simulink model "D53_LKA_Software"  (R2018b)
settings: Solver=ode3  StartTime=0.0  StopTime=10.0  FixedStep=0.01  RelTol=1e-3  EnableMultiTasking=on
model workspace (MAT data in the model file):
  MCOS : class17 (value not decoded)
  MCOS : class17 (value not decoded)
  MCOS : class17 (value not decoded)
  MCOS : class17 (value not decoded)
  MCOS : class17 (value not decoded)
  MCOS : class17 (value not decoded)
  MCOS : class17 (value not decoded)
  MCOS : class17 (value not decoded)
  MCOS : class17 (value not decoded)
  MCOS : class17 (value not decoded)
  MCOS : class17 (value not decoded)
  MCOS : class17 (value not decoded)
  MCOS : class17 (value not decoded)
  MCOS : class17 (value not decoded)
  MCOS : class17 (value not decoded)
  MCOS : class17 (value not decoded)
  MCOS : class17 (value not decoded)
  MCOS : class17 (value not decoded)
  MCOS : class17 (value not decoded)
  MCOS : class17 (value not decoded)
  MCOS : class17 (value not decoded)
  MCOS : class17 (value not decoded)
  MCOS : class17 (value not decoded)
  MCOS : class17 (value not decoded)
  MCOS : class17 (value not decoded)
  MCOS : class17 (value not decoded)
  MCOS : class17 (value not decoded)
  MCOS : class17 (value not decoded)
  MCOS : class17 (value not decoded)
  MCOS : class17 (value not decoded)
  MCOS : class17 (value not decoded)
  MCOS : class17 (value not decoded)
  MCOS : class17 (value not decoded)
  MCOS : class17 (value not decoded)
  MCOS : class17 (value not decoded)
  MCOS : class17 (value not decoded)
  MCOS : class17 (value not decoded)
  MCOS : class17 (value not decoded)
  MCOS : class17 (value not decoded)
  MCOS : class17 (value not decoded)
  MCOS : class17 (value not decoded)
  MCOS : class17 (value not decoded)
  MCOS : class17 (value not decoded)
  MCOS : class17 (value not decoded)
  MCOS : class17 (value not decoded)
  MCOS : class17 (value not decoded)
  MCOS : class17 (value not decoded)
  MCOS : class17 (value not decoded)
  MCOS : class17 (value not decoded)
  MCOS : class17 (value not decoded)
  MCOS : class17 (value not decoded)
  MCOS : class17 (value not decoded)
  MCOS : class17 (value not decoded)
  MCOS : class17 (value not decoded)
  MCOS : class17 (value not decoded)
  MCOS : class17 (value not decoded)
  MCOS : class17 (value not decoded)
  MCOS : class17 (value not decoded)
  MCOS : class17 (value not decoded)
  MCOS : class17 (value not decoded)
  MCOS : class17 (value not decoded)
  MCOS : class17 (value not decoded)
  MCOS : class17 (value not decoded)
  MCOS : class17 (value not decoded)
  MCOS : class17 (value not decoded)
  MCOS : class17 (value not decoded)
  MCOS : class17 (value not decoded)
  MCOS : class17 (value not decoded)
  MCOS : class17 (value not decoded)
  MCOS : class17 (value not decoded)
  MCOS : class17 (value not decoded)
  MCOS : class17 (value not decoded)
  MCOS : class17 (value not decoded)
  MCOS : class17 (value not decoded)
  MCOS : class17 (value not decoded)
  MCOS : class17 (value not decoded)
  MCOS : class17 (value not decoded)
  MCOS : class17 (value not decoded)
  MCOS : class17 (value not decoded)
  MCOS : class17 (value not decoded)
  MCOS : class17 (value not decoded)
  MCOS : class17 (value not decoded)
  MCOS : class17 (value not decoded)
  MCOS : class17 (value not decoded)
  MCOS : class17 (value not decoded)
  MCOS : class17 (value not decoded)
  MCOS : class17 (value not decoded)
  MCOS : class17 (value not decoded)
  MCOS : class17 (value not decoded)
undefined symbols (not defined in the file or in its folder): LKA_CarWidth, LKA_SampleTime, LKA_StrRatio_C, LKA_Veh2CamL_C, LKA_Veh2CamW_C, LKA_WhlBaseL_C, LL_CompSWA_C, LL_CrvtPrvwT_C, LL_DesDvt_C, LL_DvtComp_C, LL_DvtPrvwT_C, LL_DvtSpdDet_vDvtSpdMin_C, LL_HdAgExT_C, LL_HdAgPrvwT_C, LL_LAccMax_C, LL_LAccRMax_C, LL_LDW_EarliestWarnLine_C, LL_LDW_LatestWarnLine_C, LL_LDWS_SUPPRESS_HEADING, LL_LFClb_TFC_DiffCtlBalance, LL_LFClb_TFC_DiffCtrlMaxSWA, LL_LFClb_TFC_DiffCtrlRatio, LL_LFClb_TFC_facmGainLutGain1_C, LL_LFClb_TFC_facmGainLutGain2_C, LL_LFClb_TFC_facmIntegRatio, LL_LFClb_TFC_facmKlat_C, LL_LFClb_TFC_FfCtlRatio_C, LL_LFClb_TFC_phiIntegCtlMaxSWA_C, LL_LFClb_TFC_tiKlatPrvwT_C, LL_LFClb_TFC_vGainLutVehSpdLwr_C, LL_LFClb_TFC_vGainLutVehSpdUpr_C, LL_LKA_EarliestWarnLine_C, LL_LKA_LatestWarnLine_C, LL_LKAExPrcs_ExitC0Dvt, LL_LKAExPrcs_ExitC0Swt, LL_LKAExPrcs_tiExitTime1, LL_LKAExPrcs_tiExitTime2, LL_LKAExPrcs_tiExitTime3, LL_LKAS_OUT_OF_CONTROL_LAT_VEL, LL_LKAS_OUT_OF_CONTROL_TTLC, LL_LKASWASyn_M0, LL_LKASWASyn_M1, LL_LKASWASyn_M2, LL_LKASWASyn_M3K, LL_LKASWASyn_SWAaddMax, LL_LKASWASyn_T2, LL_LKASWASyn_tiTrqSwaRtTime, LL_LKASWASyn_tiTrqSwaTime, LL_LKASWASyn_TrqMax, LL_LKASWASyn_TrqSwaAddSwt, LL_LKASWASyn_TrqSwaRateDiff, LL_LSpdCompT_C, LL_lStpLngth_C, LL_MAX_DELAY_EPSSTAR_TIME, LL_MAX_DRIVER_TORQUE_DISABLE, LL_MAX_DRIVER_TORQUE_ENABLE, LL_MAX_LANE_WIDTH_DISABLE, LL_MAX_LANE_WIDTH_ENABLE, LL_MAX_LAT_ACC_DISABLE, LL_MAX_LAT_ACC_ENABLE ... (+30)
libraries: simulink x167, canmsglib x52, dspstat3 x3, simulink_extras x1
(part 4 of 21)

== system D53_LKA_Software/CAN Monitor (CANMon)/Subsystem1 ==
  In1 : Inport
  In2 : Inport  Port=2
  Abs : Abs
  Add : Sum  OutDataTypeStr=single
  Compare To Zero : simulink/Logic and Bit Operations/Compare To Zero  relop===  OutDataTypeStr=boolean
  Constant : Constant  OutDataTypeStr=single  SampleTime=-1
  Constant1 : Constant  Value=0.000000001  OutDataTypeStr=single  SampleTime=-1
  Divide : Product  Inputs=*/  OutDataTypeStr=single
  Switch : Switch  Criteria=u2 ~= 0
  Out1 : Outport
  wires:
  Add/1 -> Abs/1
  In1/1 -> Add/1
  Compare To Zero/1 -> Switch/2
  In2/1 -> Add/2
  Constant/1 -> Divide/1
  Switch/1 -> Divide/2
  Constant1/1 -> Switch/1
  Divide/1 -> Out1/1
  Abs/1 -> Switch/3, Compare To Zero/1

== system D53_LKA_Software/LL/Fault_Diagnostic ==
  bsInInfo : Inport
  Bus Creator : BusCreator  Inputs=2
  Bus Creator1 : BusCreator  Inputs=12
  Bus Selector3 : BusSelector  OutputSignals=DTC_Indicator.LKAS_BSWDTC_Status
  Bus Selector4 : BusSelector  OutputSignals=bsVehMovInfo.ESC_VehSpd_Valid,bsEPSInfo.EPS_LKA_State,bsEPSInfo.EPS_Error_State,bsEPSInfo.SAS_Clb_State,bsEPSInfo.SAS_Trim_State,bsSWAInfo.SWS_Fault_Code,bsSWAInfo.SAS_In_Status,bsPTState.TCU_ActualGear,bsEPSInfo.EPS_TrqLim_State,bsEPSInfo.EPS_Trq_State,bsVehMovInfo.ESC_LatAcc_Valid,bsVehMovInfo.ESC_YawRate_Valid,bsVehMovInfo.ESC_LonAcc_Valid
  Compare To Constant26 : simulink/Logic and Bit Operations/Compare To Constant  relop=~=  const=1  OutDataTypeStr=boolean
  Compare To Constant27 : simulink/Logic and Bit Operations/Compare To Constant  relop===  const=4  OutDataTypeStr=boolean
  Compare To Constant{28,30,36..39} (6 alike) : simulink/Logic and Bit Operations/Compare To Constant  relop===  const=1  OutDataTypeStr=boolean
  Compare To Constant29 : simulink/Logic and Bit Operations/Compare To Constant  relop===  const=0  OutDataTypeStr=boolean
  Compare To Constant31 : simulink/Logic and Bit Operations/Compare To Constant  relop===  const=2  OutDataTypeStr=boolean
  Compare To Constant32 : simulink/Logic and Bit Operations/Compare To Constant  relop=~=  const=0  OutDataTypeStr=boolean
  Compare To Constant33 : simulink/Logic and Bit Operations/Compare To Constant  relop=~=  const=1  OutDataTypeStr=boolean
  Compare To Constant34 : simulink/Logic and Bit Operations/Compare To Constant  relop=>  const=3  OutDataTypeStr=boolean
  Compare To Constant35 : simulink/Logic and Bit Operations/Compare To Constant  relop===  const=0  OutDataTypeStr=boolean
  Logical Operator5 : Logic  Operator=OR  AllPortsSameDT=off  OutDataTypeStr=boolean
  Logical Operator6 : Logic  Operator=OR  AllPortsSameDT=off  OutDataTypeStr=boolean
  bsSignalFault : Outport
  wires:
  Bus Creator/1 -> bsSignalFault/1
  Bus Selector3/1 -> Bus Creator/1  "<LKAS_BSWDTC_Status>"
  bsInInfo/1 -> Bus Selector4/1, Bus Selector3/1
  Bus Selector4/1 -> Compare To Constant26/1  "<ESC_VehSpd_Valid>"
  Compare To Constant26/1 -> Bus Creator1/1  "Event_FaulVehSpeed"
  Bus Selector4/2 -> Compare To Constant27/1  "<EPS_LKA_State>"
  Bus Selector4/4 -> Compare To Constant29/1  "<SAS_Clb_State>"
  Compare To Constant29/1 -> Bus Creator1/4  "Event_FaulSASClb"
  Bus Selector4/5 -> Compare To Constant30/1  "<SAS_Trim_State>"
  Bus Selector4/6 -> Compare To Constant32/1  "<SWS_Fault_Code>"
  Bus Selector4/7 -> Compare To Constant33/1  "<SAS_In_Status>"
  Bus Selector4/8 -> Compare To Constant34/1  "<TCU_ActualGear>"
  Bus Selector4/9 -> Compare To Constant35/1  "<EPS_TrqLim_State>"
  Bus Selector4/10 -> Compare To Constant36/1  "<EPS_Trq_State>"
  Bus Selector4/11 -> Compare To Constant37/1  "<ESC_LatAcc_Valid>"
  Bus Selector4/12 -> Compare To Constant38/1  "<ESC_YawRate_Valid>"
  Bus Selector4/13 -> Compare To Constant39/1  "<ESC_LonAcc_Valid>"
  Compare To Constant30/1 -> Bus Creator1/5  "Event_FaulSASTrim"
  Compare To Constant31/1 -> Logical Operator5/2
  Compare To Constant28/1 -> Logical Operator5/1
  Bus Selector4/3 -> Compare To Constant31/1, Compare To Constant28/1  "<EPS_Error_State>"
  Compare To Constant32/1 -> Logical Operator6/1
  Compare To Constant33/1 -> Logical Operator6/2
  Compare To Constant35/1 -> Bus Creator1/8  "Event_FaulTrqLim"
  Compare To Constant34/1 -> Bus Creator1/7  "Event_FaulTCUGear"
  Compare To Constant36/1 -> Bus Creator1/9  "Event_FaulEPSTrqSt"
  Compare To Constant37/1 -> Bus Creator1/10  "Event_FaulLatAcc"
  Compare To Constant38/1 -> Bus Creator1/11  "Event_FaulYawRate"
  Compare To Constant39/1 -> Bus Creator1/12  "Event_FaulLonAcc"
  Bus Creator1/1 -> Bus Creator/2  "LKAS_ASWDTC_Status"
  Compare To Constant27/1 -> Bus Creator1/2  "Event_FaulEPSLKASt"
  Logical Operator5/1 -> Bus Creator1/3  "Event_FaulETATDA"
  Logical Operator6/1 -> Bus Creator1/6  "Event_FaulSWS"

== system D53_LKA_Software/LL/Human Machine Interface (HMI) ==
  HMI_stDACmode : Inport
  HMI_LDWWarn : Inport  Port=2
  HMI_LKA_STATE : Inport  Port=3
  HMI_LDW_STATE : Inport  Port=4
  HMI_R0_Quality : Inport  Port=5
  HMI_L0_Quality : Inport  Port=6
  HMI_EPSInfo : Inport  Port=7
  HMI_camera_common_fault : Inport  Port=8
  HMI_Front_Camera_Blocked : Inport  Port=9
  HMI_stFaultCSyn : Inport  Port=10
  Bus Creator2 : BusCreator  Inputs=7
  Cast To Single{,1..6} (7 alike) : DataTypeConversion  OutDataTypeStr=uint8
  HMI_Popup_Status : MATLAB Function  TreatAsAtomicUnit=on
  Hands_off_warning : MATLAB Function  TreatAsAtomicUnit=on
  LDW_Flag : MATLAB Function  TreatAsAtomicUnit=on
  LDW_Status_Display : MATLAB Function  TreatAsAtomicUnit=on
  LKA_Status_Display : MATLAB Function  TreatAsAtomicUnit=on
  LKA_action_indication : MATLAB Function  TreatAsAtomicUnit=on
  Subsystem : Subsystem
  Vehicle_Lane_Display : MATLAB Function  TreatAsAtomicUnit=on
  HMI_LDWLKA : Outport
  wires:
  HMI_LKA_STATE/1 -> Vehicle_Lane_Display/2(LKA_STATE), LKA_Status_Display/2(LKA_STATE), LDW_Flag/2(HMI_LKA_STATE), HMI_Popup_Status/2(LKA_STATE), LKA_action_indication/2(LKA_STATE)  "HMI_LKA_STATE"
  HMI_LDW_STATE/1 -> Subsystem/1(LDW_STATE), Vehicle_Lane_Display/3(LDW_STATE), LDW_Status_Display/2(LDW_STATE)  "HMI_LDW_STATE"
  Hands_off_warning/1(Hands_off_warning) -> Cast To Single4/1  "Hands_off_warning"
  LDW_Status_Display/1(LDW_Status_Display) -> Cast To Single1/1  "LDW_Status_Display"
  HMI_stFaultCSyn/1 -> HMI_Popup_Status/6(stFaultCSyn)  "HMI_stFaultCSyn"
  Bus Creator2/1 -> HMI_LDWLKA/1
  HMI_L0_Quality/1 -> Vehicle_Lane_Display/5(L0_Quality)  "HMI_L0_Quality"
  HMI_Popup_Status/1(HMI_Popup_Status) -> Cast To Single6/1  "HMI_Popup_Status"
  LKA_Status_Display/1(LKA_Status_Display) -> Cast To Single2/1  "LKA_Status_Display"
  HMI_stDACmode/1 -> Vehicle_Lane_Display/1(stDACmode), LDW_Status_Display/1(stDACmode), HMI_Popup_Status/1(stDACmode), LKA_action_indication/1(stDACmode), LDW_Flag/1(HMI_stDACmode), LKA_Status_Display/1(stDACmode)  "HMI_stDACmode"
  LDW_Flag/1(LDW_Flag) -> Cast To Single3/1  "LDW_Flag"
  HMI_Front_Camera_Blocked/1 -> HMI_Popup_Status/5(Front_Camera_Blocked)  "HMI_Front_Camera_Blocked"
  HMI_R0_Quality/1 -> Vehicle_Lane_Display/4(R0_Quality)  "HMI_R0_Quality"
  HMI_camera_common_fault/1 -> HMI_Popup_Status/4(camera_common_fault)  "HMI_camera_common_fault"
  LKA_action_indication/1(LKA_action_indication) -> Cast To Single5/1  "LKA_action_indication"
  Vehicle_Lane_Display/1(Vehicle_Lane_Display) -> Cast To Single/1  "Vehicle_Lane_Display"
  Cast To Single/1 -> Bus Creator2/1  "Vehicle_Lane_Display"
  Cast To Single1/1 -> Bus Creator2/2  "LDW_Status_Display"
  Cast To Single2/1 -> Bus Creator2/3  "LKA_Status_Display"
  Cast To Single3/1 -> Bus Creator2/4  "LDW_Flag"
  Cast To Single4/1 -> Bus Creator2/5  "Hands_off_warning"
  Cast To Single5/1 -> Bus Creator2/6  "LKA_action_indication"
  Cast To Single6/1 -> Bus Creator2/7  "HMI_Popup_Status"
  HMI_EPSInfo/1 -> Subsystem/2(EPSInfo)  "HMI_EPSInfo"
  Subsystem/1(HandsOff10s) -> HMI_Popup_Status/3(HandsOff)
  Subsystem/2(HandsOff15s) -> Hands_off_warning/1(HandsOff)
  HMI_LDWWarn/1 -> LDW_Flag/3(HMI_LDWWarnInfo)

== system D53_LKA_Software/LL/LL Inputs Mapping ==
  bsInInfo : Inport
  Bus Creator : BusCreator  Inputs=7
  Bus Selector : BusSelector  OutputSignals=bsMP5Info,bsLaneInfo,bsEPSInfo,bsVehMovInfo,bsSWAInfo,bsBCMInfo,bsPTState
  bsBCMInfo : Subsystem
  bsEPSInfo : Subsystem
  bsLaneInfo : Subsystem
  bsMP5Info : Subsystem
  bsPTState : Subsystem
  bsSWAInfo : Subsystem
  bsVehMovInfo : Subsystem
  bsInfo : Outport
  wires:
  bsInInfo/1 -> Bus Selector/1
  Bus Creator/1 -> bsInfo/1
  Bus Selector/2 -> bsLaneInfo/1(bsLaneInfoIn)  "<bsLaneInfo>"
  Bus Selector/3 -> bsEPSInfo/1(bsEPSInfoIn)  "<bsEPSInfo>"
  bsEPSInfo/1(bsEPSInfoOut) -> Bus Creator/3  "bsEPSInfo"
  Bus Selector/4 -> bsVehMovInfo/1(bsVehMovInfoIn)  "<bsVehMovInfo>"
  bsVehMovInfo/1(bsVehMovInfoOut) -> Bus Creator/4  "bsVehMovInfo"
  Bus Selector/5 -> bsSWAInfo/1(bsSWAInfoIn)  "<bsSWAInfo>"
  Bus Selector/6 -> bsBCMInfo/1(bsBCMInfoIn)  "<bsBCMInfo>"
  Bus Selector/1 -> bsMP5Info/1(bsMP5InfoIn)  "<bsMP5Info>"
  bsMP5Info/1(bsMP5InfoOut) -> Bus Creator/1  "bsMP5Info"
  bsBCMInfo/1(bsBCMInfoOut) -> Bus Creator/6  "bsBCMInfo"
  Bus Selector/7 -> bsPTState/1(bsPTStateIn)  "<bsPTState>"
  bsPTState/1(bsPTStateOut) -> Bus Creator/7  "bsPTState"
  bsLaneInfo/1(bsLaneInfoOut) -> Bus Creator/2  "bsLaneInfo"
  bsSWAInfo/1(bsSWAInfoOut) -> Bus Creator/5  "bsSWAInfo"

== system D53_LKA_Software/LL/LL Output (LLOut) ==
  LLOut_bsLLState : Inport
  LLOut_phiSWACmd : Inport  Port=2
  LLOut_bsLLHMI : Inport  Port=3
  LLOut_M : Inport  Port=4
  Bus Creator : BusCreator  Inputs=15
  Bus Selector1 : BusSelector  OutputSignals=LKA_State,DACMode
  Bus Selector2 : BusSelector  OutputSignals=Vehicle_Lane_Display,LDW_Status_Display,LKA_Status_Display,LDW_Flag,Hands_off_warning,LKA_action_indication,HMI_Popup_Status
  Cast To Single : DataTypeConversion  OutDataTypeStr=single
  Cast To Single{2,4..15} (13 alike) : DataTypeConversion  OutDataTypeStr=uint8
  Cast To Single3 : DataTypeConversion  OutDataTypeStr=single
  Compare To Constant : simulink/Logic and Bit Operations/Compare To Constant  relop===  const=4  OutDataTypeStr=boolean
  Compare To Constant1 : simulink/Logic and Bit Operations/Compare To Constant  relop=>  const=0  OutDataTypeStr=boolean
  Constant : Constant  Value=0  OutDataTypeStr=uint8
  Constant1 : Constant  OutDataTypeStr=uint8
  Constant15 : Constant  Value=0  OutDataTypeStr=uint16
  Constant2 : Constant  Value=2  OutDataTypeStr=uint8
  Constant25 : Constant  Value=0  OutDataTypeStr=uint8
  Constant26 : Constant  Value=0  OutDataTypeStr=uint8
  Constant3 : Constant  Value=3  OutDataTypeStr=uint8
  Constant4 : Constant  Value=4  OutDataTypeStr=uint8
  Constant5 : Constant  Value=4  OutDataTypeStr=uint8
  Constant6 : Constant  Value=5  OutDataTypeStr=uint8
  Constant7 : Constant  Value=0  OutDataTypeStr=single
  Multiport Switch : MultiPortSwitch  DataPortOrder=Zero-based contiguous  Inputs=7  zeroidx=on
  Switch : Switch  Criteria=u2 > Threshold
  LL_bsLLOut : Outport
  wires:
  Constant/1 -> Multiport Switch/2
  Constant5/1 -> Multiport Switch/7
  Cast To Single13/1 -> Bus Creator/13  "LKA_Mode_from_Camera"
  Cast To Single11/1 -> Bus Creator/11  "Hands_off_warning"
  Constant25/1 -> Cast To Single14/1  "TJA_HMI_Txt_Disp"
  LLOut_M/1 -> Switch/1
  Bus Selector2/2 -> [LDW_Status_Display]  "<LDW_Status_Display>"
  Cast To Single9/1 -> Bus Creator/9  "HMI_Popup_Status"
  Constant4/1 -> Multiport Switch/6
  Bus Selector2/6 -> [LKA_action_indication]  "<LKA_action_indication>"
  Cast To Single15/1 -> Bus Creator/15  "TJA_status_icon"
  Compare To Constant1/1 -> [LKA_Switch_State]
  LLOut_bsLLState/1 -> Bus Selector1/1
  Constant1/1 -> Multiport Switch/3
  Bus Selector2/1 -> [Vehicle_Lane_Display]  "<Vehicle_Lane_Display>"
  LLOut_bsLLHMI/1 -> Bus Selector2/1
  [EPS_State_Ctl] -> Cast To Single2/1  "EPS_State_Ctl"
  [LKA_Mode_from_Camera] -> Cast To Single13/1  "LKA_Mode_from_Camera"
  Cast To Single12/1 -> Bus Creator/12  "Vehicle_Lane_Display"
  Cast To Single6/1 -> Bus Creator/6  "LDW_Status_Display"
  Constant7/1 -> Switch/3
  Switch/1 -> [Coefficient_toregulate_EPS]  "Coefficient_toregulate_EPS"
  Multiport Switch/1 -> [EPS_State_Ctl], Compare To Constant/1  "EPS_State_Ctl"
  Bus Selector2/5 -> [Hands_off_warning]  "<Hands_off_warning>"
  Constant3/1 -> Multiport Switch/5
  Cast To Single3/1 -> Bus Creator/3  "Coefficient_toregulate_EPS"
  Cast To Single14/1 -> Bus Creator/14  "TJA_HMI_Txt_Disp"
  Bus Creator/1 -> LL_bsLLOut/1  "LL_bsLLOut"
  Cast To Single2/1 -> Bus Creator/2  "EPS_State_Ctl"
  Constant2/1 -> Multiport Switch/4
  Bus Selector1/2 -> [LKA_Mode_from_Camera], Compare To Constant1/1  "<DACMode>"
  Cast To Single10/1 -> Bus Creator/10  "LKA_Switch_State"
  Cast To Single4/1 -> Bus Creator/4  "Permit_to_know_if_LKA_or_LPA3F2"
  Cast To Single8/1 -> Bus Creator/8  "LKA_Status_Display"
  Constant26/1 -> Cast To Single15/1  "TJA_status_icon"
  [Hands_off_warning] -> Cast To Single11/1  "Hands_off_warning"
  [LKA_Switch_State] -> Cast To Single10/1  "LKA_Switch_State"
  [LDW_Status_Display] -> Cast To Single6/1  "LDW_Status_Display"
  Cast To Single/1 -> Bus Creator/1  "LMS_phiSWACmd"
  Bus Selector2/3 -> [LKA_Status_Display]  "<LKA_Status_Display>"
  LLOut_phiSWACmd/1 -> Cast To Single/1  "LMS_phiSWACmd"
  Bus Selector2/4 -> [LDW_Flag]  "<LDW_Flag>"
  [LKA_Status_Display] -> Cast To Single8/1  "LKA_Status_Display"
  Bus Selector1/1 -> Multiport Switch/1  "<LKA_State>"
  [HMI_Popup_Status] -> Cast To Single9/1  "HMI_Popup_Status"
  Cast To Single5/1 -> Bus Creator/5  "LDW_Flag"
  Constant6/1 -> Multiport Switch/8
  [LKA_action_indication] -> Cast To Single7/1  "LKA_action_indication"
  [Coefficient_toregulate_EPS] -> Cast To Single3/1  "Coefficient_toregulate_EPS"
  [LDW_Flag] -> Cast To Single5/1  "LDW_Flag"
  Constant15/1 -> Cast To Single4/1  "Permit_to_know_if_LKA_or_LPA3F2"
  [Vehicle_Lane_Display] -> Cast To Single12/1  "Vehicle_Lane_Display"
  Compare To Constant/1 -> Switch/2
  Bus Selector2/7 -> [HMI_Popup_Status]  "<HMI_Popup_Status>"
  Cast To Single7/1 -> Bus Creator/7  "LKA_action_indication"

== system D53_LKA_Software/LL/LLOn ==
  stDACMode : Inport
  bsInInfo : Inport  Port=2
  bsLLClb : Inport  Port=3
  bsSignalFault : Inport  Port=4
  states : EnablePort  StatesWhenEnabling=reset
      settings: AttributesFormatString=states = %<StatesWhenEnabling>
  Bus Selector : BusSelector  OutputSignals=bsLLSMConClb,bsLDWClb,bsLKAClb,bsConstantClb
  LDW : Subsystem  Description=|  TreatAsAtomicUnit=on
      | Block Name: Lane Departure Warning
      | Ab.: LDW
      | No.: 1.3.0.0
      | Rev: 0.0.1
      | Update Date: 19-3-26
  LKA : Subsystem  Description=|  TreatAsAtomicUnit=on
      | Block Name: Lane Keeping Assistance
      | Ab.: LKA
      | No.: 1.2.0.0
      | Rev: 0.0.1
      | Update Date: 19-5-13
  LKA Input Processing (LKAInP) : Subsystem
  LL State Determination (LLStateDet) : Subsystem
  bsLLState : Outport  OutputWhenDisabled=reset  InitialOutput=0
  LDW_Flag : Outport  Port=2
  phiSWACmd : Outport  Port=3  OutputWhenDisabled=reset  InitialOutput=0
  M : Outport  Port=4  OutputWhenDisabled=reset  InitialOutput=0
  tag scope: LLClb_bsConstantClb=global, LLClb_bsLDWClb=global, LLClb_bsLKAClb=global, LLClb_bsLLSMConClb=global
  wires:
  [ActFlg] -> LKA Input Processing (LKAInP)/1(LKAInP_stLKAActvFlg)
  LL State Determination (LLStateDet)/2(LLStateDet_stLDWActvFlg) -> LDW/Enable, LDW/1(LDW_stLDWActvFlg)
  [LLClb_bsLLSMConClb] -> LL State Determination (LLStateDet)/4(LLStateDet_bsLLSMConClb)
  [LLClb_bsLKAClb] -> LKA Input Processing (LKAInP)/3(LKAInP_bsLKAClb)
  LL State Determination (LLStateDet)/1(LLStateDet_bsLLState) -> bsLLState/1
  [LLClb_bsLDWClb] -> LDW/3(LDW_bsLDWClb)
  LKA Input Processing (LKAInP)/1(LKAInP_bsLKAInPInfo) -> LKA/2(LKA_bsLKAInPInfo), LL State Determination (LLStateDet)/3(LLStateDet_bsLKAInPInfo)
  bsLLClb/1 -> Bus Selector/1
  [LLClb_bsLKAClb] -> LKA/3(LKA_bsLKAClb)
  Bus Selector/1 -> [LLClb_bsLLSMConClb]  "<bsLLSMConClb>"
  stDACMode/1 -> LL State Determination (LLStateDet)/1(LLStateDet_stDACMode)
  Bus Selector/3 -> [LLClb_bsLKAClb]  "<bsLKAClb>"
  Bus Selector/2 -> [LLClb_bsLDWClb]  "<bsLDWClb>"
  LL State Determination (LLStateDet)/3(LLStateDet_stLKAActvFlg) -> [ActFlg], LKA/Enable
  LDW/1(LDW_Flag) -> LDW_Flag/1  "LDW_Flag"
  bsInInfo/1 -> LKA Input Processing (LKAInP)/2(LKAInP_bsInInfoSyn), LL State Determination (LLStateDet)/2(LLStateDet_bsInInfoSyn), LKA/1(LKA_bsInInfoSyn), LDW/2(LDW_bsInInfoSyn)
  [ExitFlg] -> LL State Determination (LLStateDet)/5(LLStateDet_stExitFlg)
  Bus Selector/4 -> [LLClb_bsConstantClb]  "<bsConstantClb>"
  [LLClb_bsConstantClb] -> LKA/4(LKA_bsConstantClb)
  LKA/2(LKA_phiSWACmd) -> phiSWACmd/1  "OutputSWACmd"
  LKA/1(LKA_ExitFlg) -> [ExitFlg]
  bsSignalFault/1 -> LL State Determination (LLStateDet)/6(LLStateDet_SignalFault)
  LKA/3(LKA_M) -> M/1  "OutputM"

== system D53_LKA_Software/LL/Subsystem ==
  bsInfo : Inport
  Bus Selector : BusSelector  OutputSignals=bsMP5Info.LKA_Main_Switch,bsMP5Info.LKA_Mode
  On : Outport  OutDataTypeStr=uint8
  Mode : Outport  Port=2  OutDataTypeStr=uint8
  wires:
  Bus Selector/2 -> Mode/1  "<LKA_Mode>"
  bsInfo/1 -> Bus Selector/1
  Bus Selector/1 -> On/1  "<LKA_Main_Switch>"

== system D53_LKA_Software/LLClb/ConstantClb ==
  Bus Creator : BusCreator  Inputs=6
  Data Type Conversion{2..4,6,13,22} (6 alike) : DataTypeConversion  OutDataTypeStr=single
  LKA_CarWidth=1.8 : Constant  Value=LKA_CarWidth
  LKA_SampleTime=0.01 : Constant  Value=LKA_SampleTime  OutDataTypeStr=single
  LKA_StrRatio_C=15.3 : Constant  Value=LKA_StrRatio_C
  LKA_Veh2CamL_C=1.56 : Constant  Value=LKA_Veh2CamL_C
  LKA_Veh2CamW_C=0.9 : Constant  Value=LKA_Veh2CamW_C  OutDataTypeStr=single
  LKA_WhlBaseL_C=2.65 : Constant  Value=LKA_WhlBaseL_C
  Switch{,1..3,11,19} (6 alike) : Switch  Criteria=u2 ~= 0  OutDataTypeStr=single
  ConstantClb : Outport
  wires:
  LKA_Veh2CamW_C=0.9/1 -> Switch/3  "LKA_Veh2CamW_C"
  Data Type Conversion13/1 -> Switch/1, Switch/2
  Data Type Conversion2/1 -> Switch1/1, Switch1/2
  LKA_Veh2CamL_C=1.56/1 -> Switch1/3  "LKA_Veh2CamL_C"
  LKA_WhlBaseL_C=2.65/1 -> Switch2/3  "LKA_WhlBaseL_C"
  Data Type Conversion4/1 -> Switch2/1, Switch2/2
  Data Type Conversion6/1 -> Switch3/1, Switch3/2
  LKA_StrRatio_C=15.3/1 -> Switch3/3  "LKA_StrRatio_C"
  Data Type Conversion22/1 -> Switch11/1, Switch11/2
  LKA_CarWidth=1.8/1 -> Switch11/3  "LKA_CarWidth"
  Bus Creator/1 -> ConstantClb/1
  Switch3/1 -> Bus Creator/5  "LKA_StrRatio_C"
  Switch11/1 -> Bus Creator/6  "LKA_CarWidth"
  Switch1/1 -> Bus Creator/3  "LKA_Veh2CamL_C"
  Switch/1 -> Bus Creator/2  "LKA_Veh2CamW_C"
  Switch2/1 -> Bus Creator/4  "LKA_WhlBaseL_C"
  Switch19/1 -> Bus Creator/1  "LKA_SampleTime"
  Data Type Conversion3/1 -> Switch19/2, Switch19/1
  LKA_SampleTime=0.01/1 -> Switch19/3  "LKA_SampleTime"

== system D53_LKA_Software/LLClb/LDWClb ==
  Bus Creator : BusCreator  Inputs=1
  Data Type Conversion6 : DataTypeConversion  OutDataTypeStr=single
  LL_LDWS_SUPPRESS_HEADING=2 : Constant  Value=LL_LDWS_SUPPRESS_HEADING  OutDataTypeStr=single
  Switch2 : Switch  Criteria=u2 ~= 0  OutDataTypeStr=single
  LDWClb : Outport
  wires:
  Bus Creator/1 -> LDWClb/1
  Switch2/1 -> Bus Creator/1  "LL_LDWS_SUPPRESS_HEADING"
  LL_LDWS_SUPPRESS_HEADING=2/1 -> Switch2/3
  Data Type Conversion6/1 -> Switch2/1, Switch2/2

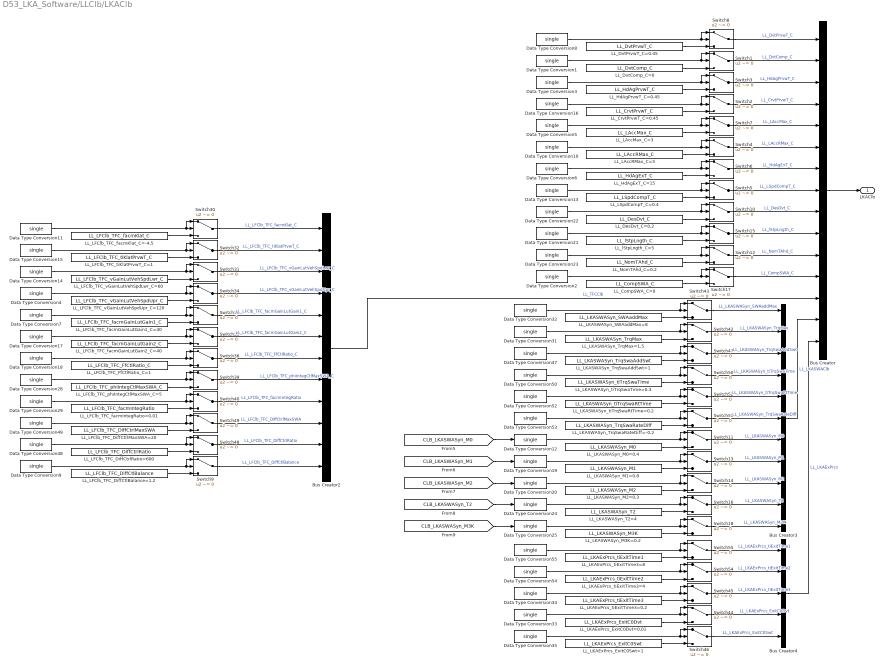
== system D53_LKA_Software/LLClb/LKAClb ==
  Bus Creator : BusCreator  Inputs=15
  Bus Creator2 : BusCreator  Inputs=12
  Bus Creator3 : BusCreator  Inputs=11
  Bus Creator4 : BusCreator  Inputs=5
  Data Type Conversion{1..25,28..29,31..35,47..50,52..55} (40 alike) : DataTypeConversion  OutDataTypeStr=single
  LL_CompSWA_C=0 : Constant  Value=LL_CompSWA_C  OutDataTypeStr=single
  LL_CrvtPrvwT_C=0.45 : Constant  Value=LL_CrvtPrvwT_C  OutDataTypeStr=single
  LL_DesDvt_C=0.2 : Constant  Value=LL_DesDvt_C  OutDataTypeStr=single
  LL_DvtComp_C=0 : Constant  Value=LL_DvtComp_C  OutDataTypeStr=single
  LL_DvtPrvwT_C=0.45 : Constant  Value=LL_DvtPrvwT_C  OutDataTypeStr=single
  LL_HdAgExT_C=15 : Constant  Value=LL_HdAgExT_C  OutDataTypeStr=single
  LL_HdAgPrvwT_C=0.45 : Constant  Value=LL_HdAgPrvwT_C  OutDataTypeStr=single
  LL_LAccMax_C=3 : Constant  Value=LL_LAccMax_C  OutDataTypeStr=single
  LL_LAccRMax_C=5 : Constant  Value=LL_LAccRMax_C  OutDataTypeStr=single
  LL_LFClb_TFC_DiffCtlBalance=1.2 : Constant  Value=LL_LFClb_TFC_DiffCtlBalance  OutDataTypeStr=single
  LL_LFClb_TFC_DiffCtrlMaxSWA=20 : Constant  Value=LL_LFClb_TFC_DiffCtrlMaxSWA  OutDataTypeStr=single
  LL_LFClb_TFC_DiffCtrlRatio=600 : Constant  Value=LL_LFClb_TFC_DiffCtrlRatio  OutDataTypeStr=single
  LL_LFClb_TFC_FfCtlRatio_C=1 : Constant  Value=LL_LFClb_TFC_FfCtlRatio_C  OutDataTypeStr=single
  LL_LFClb_TFC_facmGainLutGain1_C=40 : Constant  Value=LL_LFClb_TFC_facmGainLutGain1_C  OutDataTypeStr=single
  LL_LFClb_TFC_facmGainLutGain2_C=40 : Constant  Value=LL_LFClb_TFC_facmGainLutGain2_C  OutDataTypeStr=single
  LL_LFClb_TFC_facmIntegRatio=0.01 : Constant  Value=LL_LFClb_TFC_facmIntegRatio  OutDataTypeStr=single
  LL_LFClb_TFC_facmKlat_C=-4.5 : Constant  Value=LL_LFClb_TFC_facmKlat_C  OutDataTypeStr=single
  LL_LFClb_TFC_phiIntegCtlMaxSWA_C=5 : Constant  Value=LL_LFClb_TFC_phiIntegCtlMaxSWA_C  OutDataTypeStr=single
  LL_LFClb_TFC_tiKlatPrvwT_C=1 : Constant  Value=LL_LFClb_TFC_tiKlatPrvwT_C  OutDataTypeStr=single
  LL_LFClb_TFC_vGainLutVehSpdLwr_C=60 : Constant  Value=LL_LFClb_TFC_vGainLutVehSpdLwr_C  OutDataTypeStr=single
  LL_LFClb_TFC_vGainLutVehSpdUpr_C=120 : Constant  Value=LL_LFClb_TFC_vGainLutVehSpdUpr_C  OutDataTypeStr=single
  LL_LKAExPrcs_ExitC0Dvt=0.01 : Constant  Value=LL_LKAExPrcs_ExitC0Dvt  OutDataTypeStr=single
  LL_LKAExPrcs_ExitC0Swt=1 : Constant  Value=LL_LKAExPrcs_ExitC0Swt  OutDataTypeStr=single
  LL_LKAExPrcs_tiExitTime3=0.2 : Constant  Value=LL_LKAExPrcs_tiExitTime3  OutDataTypeStr=single
  LL_LKAExPrcs_tiExitTime3=4 : Constant  Value=LL_LKAExPrcs_tiExitTime2  OutDataTypeStr=single
  LL_LKAExPrcs_tiExitTime3=8 : Constant  Value=LL_LKAExPrcs_tiExitTime1  OutDataTypeStr=single
  LL_LKASWASyn_M0=0.4 : Constant  Value=LL_LKASWASyn_M0  OutDataTypeStr=single
  LL_LKASWASyn_M1=0.8 : Constant  Value=LL_LKASWASyn_M1  OutDataTypeStr=single
  LL_LKASWASyn_M2=0.3 : Constant  Value=LL_LKASWASyn_M2  OutDataTypeStr=single
  LL_LKASWASyn_M3K=0.2 : Constant  Value=LL_LKASWASyn_M3K  OutDataTypeStr=single
  LL_LKASWASyn_SWAaddMax=8 : Constant  Value=LL_LKASWASyn_SWAaddMax  OutDataTypeStr=single
  LL_LKASWASyn_T2=4 : Constant  Value=LL_LKASWASyn_T2  OutDataTypeStr=single
  LL_LKASWASyn_TrqMax=1.5 : Constant  Value=LL_LKASWASyn_TrqMax  OutDataTypeStr=single
  LL_LKASWASyn_TrqSwaAddSwt=1 : Constant  Value=LL_LKASWASyn_TrqSwaAddSwt  OutDataTypeStr=single
  LL_LKASWASyn_TrqSwaRateDiff=-0.2 : Constant  Value=LL_LKASWASyn_TrqSwaRateDiff  OutDataTypeStr=single
  LL_LKASWASyn_tiTrqSwaRtTime=0.2 : Constant  Value=LL_LKASWASyn_tiTrqSwaRtTime  OutDataTypeStr=single
  LL_LKASWASyn_tiTrqSwaTime=0.3 : Constant  Value=LL_LKASWASyn_tiTrqSwaTime  OutDataTypeStr=single
  LL_LSpdCompT_C=0.4 : Constant  Value=LL_LSpdCompT_C  OutDataTypeStr=single
  LL_NomTAhd_C=0.2 : Constant  Value=LL_NomTAhd_C  OutDataTypeStr=single
  LL_lStpLngth_C=5 : Constant  Value=LL_lStpLngth_C  OutDataTypeStr=single
  Switch{1..18,30..36,39..40,42..50,52..55} (40 alike) : Switch  Criteria=u2 ~= 0  OutDataTypeStr=single
  LKAClb : Outport
  wires:
  Bus Creator/1 -> LKAClb/1
  Switch8/1 -> Bus Creator/1  "LL_DvtPrvwT_C"
  Switch1/1 -> Bus Creator/2  "LL_DvtComp_C"
  Switch3/1 -> Bus Creator/3  "LL_HdAgPrvwT_C"
  Switch17/1 -> Bus Creator/12  "LL_CompSWA_C"
  Switch6/1 -> Bus Creator/7  "LL_HdAgExT_C"
  Switch7/1 -> Bus Creator/5  "LL_LAccMax_C"
  Switch4/1 -> Bus Creator/6  "LL_LAccRMax_C"
  Switch5/1 -> Bus Creator/8  "LL_LSpdCompT_C"
  Switch2/1 -> Bus Creator/4  "LL_CrvtPrvwT_C"
  Switch15/1 -> Bus Creator/10  "LL_lStpLngth_C"
  Switch10/1 -> Bus Creator/9  "LL_DesDvt_C"
  Switch12/1 -> Bus Creator/11  "LL_NomTAhd_C"
  LL_DvtPrvwT_C=0.45/1 -> Switch8/3
  Data Type Conversion8/1 -> Switch8/1, Switch8/2
  Data Type Conversion1/1 -> Switch1/2, Switch1/1
  LL_DvtComp_C=0/1 -> Switch1/3
  LL_CrvtPrvwT_C=0.45/1 -> Switch2/3
  Data Type Conversion16/1 -> Switch2/2, Switch2/1
  Data Type Conversion3/1 -> Switch3/2, Switch3/1
  LL_HdAgPrvwT_C=0.45/1 -> Switch3/3
  LL_HdAgExT_C=15/1 -> Switch6/3
  Data Type Conversion6/1 -> Switch6/2, Switch6/1
  Data Type Conversion13/1 -> Switch5/2, Switch5/1
  LL_LSpdCompT_C=0.4/1 -> Switch5/3
  LL_LAccRMax_C=5/1 -> Switch4/3
  Data Type Conversion10/1 -> Switch4/1, Switch4/2
  Data Type Conversion5/1 -> Switch7/2, Switch7/1
  LL_LAccMax_C=3/1 -> Switch7/3
  Data Type Conversion21/1 -> Switch15/2, Switch15/1
  Data Type Conversion23/1 -> Switch12/2, Switch12/1
  Data Type Conversion22/1 -> Switch10/2, Switch10/1
  Data Type Conversion2/1 -> Switch17/2, Switch17/1
  LL_DesDvt_C=0.2/1 -> Switch10/3
  LL_lStpLngth_C=5/1 -> Switch15/3
  LL_NomTAhd_C=0.2/1 -> Switch12/3
  LL_CompSWA_C=0/1 -> Switch17/3
  Bus Creator2/1 -> Bus Creator/13  "LL_TFCClb"
  Switch35/1 -> Bus Creator2/6  "LL_LFClb_TFC_facmGainLutGain2_C"
  Switch30/1 -> Bus Creator2/1  "LL_LFClb_TFC_facmKlat_C"
  Switch31/1 -> Bus Creator2/3  "LL_LFClb_TFC_vGainLutVehSpdLwr_C"
  Switch34/1 -> Bus Creator2/4  "LL_LFClb_TFC_vGainLutVehSpdUpr_C"
  Switch33/1 -> Bus Creator2/5  "LL_LFClb_TFC_facmGainLutGain1_C"
  Switch32/1 -> Bus Creator2/2  "LL_LFClb_TFC_tiKlatPrvwT_C"
  LL_LFClb_TFC_facmGainLutGain1_C=40/1 -> Switch33/3
  LL_LFClb_TFC_vGainLutVehSpdLwr_C=60/1 -> Switch31/3
  LL_LFClb_TFC_tiKlatPrvwT_C=1/1 -> Switch32/3
  Data Type Conversion11/1 -> Switch30/2, Switch30/1
  Data Type Conversion7/1 -> Switch33/2, Switch33/1
  Data Type Conversion4/1 -> Switch34/2, Switch34/1
  Data Type Conversion15/1 -> Switch32/2, Switch32/1
  Data Type Conversion17/1 -> Switch35/2, Switch35/1
  LL_LFClb_TFC_facmGainLutGain2_C=40/1 -> Switch35/3
  Data Type Conversion14/1 -> Switch31/2, Switch31/1
  LL_LFClb_TFC_vGainLutVehSpdUpr_C=120/1 -> Switch34/3
  LL_LFClb_TFC_facmKlat_C=-4.5/1 -> Switch30/3
  LL_LFClb_TFC_FfCtlRatio_C=1/1 -> Switch36/3
  Data Type Conversion18/1 -> Switch36/1, Switch36/2
  Switch36/1 -> Bus Creator2/7  "LL_LFClb_TFC_FfCtlRatio_C"
  Switch40/1 -> Bus Creator2/9  "LL_LFClb_TFC_facmIntegRatio"
  Switch39/1 -> Bus Creator2/8  "LL_LFClb_TFC_phiIntegCtlMaxSWA_C"
  LL_LFClb_TFC_phiIntegCtlMaxSWA_C=5/1 -> Switch39/3
  Data Type Conversion28/1 -> Switch39/1, Switch39/2
  LL_LFClb_TFC_facmIntegRatio=0.01/1 -> Switch40/3
  Data Type Conversion29/1 -> Switch40/1, Switch40/2
  Data Type Conversion31/1 -> Switch42/2, Switch42/1
  LL_LKASWASyn_TrqMax=1.5/1 -> Switch42/3
  LL_LKASWASyn_SWAaddMax=8/1 -> Switch43/3
  Data Type Conversion32/1 -> Switch43/1, Switch43/2
  Switch43/1 -> Bus Creator3/1  "LL_LKASWASyn_SWAaddMax"
  Switch42/1 -> Bus Creator3/2  "LL_LKASWASyn_TrqMax"
  Bus Creator3/1 -> Bus Creator/14  "LL_LKASWAClb"
  Switch44/1 -> Bus Creator4/4  "LL_LKAExPrcs_ExitC0Dvt"
  Switch45/1 -> Bus Creator4/3  "LL_LKAExPrcs_tiExitTime3"
  Data Type Conversion34/1 -> Switch45/2, Switch45/1
  LL_LKAExPrcs_tiExitTime3=0.2/1 -> Switch45/3
  LL_LKAExPrcs_ExitC0Dvt=0.01/1 -> Switch44/3
  Data Type Conversion33/1 -> Switch44/1, Switch44/2
  Bus Creator4/1 -> Bus Creator/15  "LL_LKAExPrcs"
  Data Type Conversion35/1 -> Switch46/2, Switch46/1
  LL_LKAExPrcs_ExitC0Swt=1/1 -> Switch46/3
  Switch46/1 -> Bus Creator4/5  "LL_LKAExPrcs_ExitC0Swt"
  Switch47/1 -> Bus Creator3/3  "LL_LKASWASyn_TrqSwaAddSwt"
  LL_LKASWASyn_TrqSwaAddSwt=1/1 -> Switch47/3
  Data Type Conversion47/1 -> Switch47/1, Switch47/2
  Data Type Conversion48/1 -> Switch48/2, Switch48/1
  LL_LFClb_TFC_DiffCtrlRatio=600/1 -> Switch48/3
  Switch48/1 -> Bus Creator2/11  "LL_LFClb_TFC_DiffCtrlRatio"
  Switch49/1 -> Bus Creator2/10  "LL_LFClb_TFC_DiffCtrlMaxSWA"
  LL_LFClb_TFC_DiffCtrlMaxSWA=20/1 -> Switch49/3
  Data Type Conversion49/1 -> Switch49/1, Switch49/2
  Data Type Conversion50/1 -> Switch50/2, Switch50/1
  LL_LKASWASyn_tiTrqSwaTime=0.3/1 -> Switch50/3
  Switch50/1 -> Bus Creator3/4  "LL_LKASWASyn_tiTrqSwaTime"
  Switch52/1 -> Bus Creator3/5  "LL_LKASWASyn_tiTrqSwaRtTime"
  LL_LKASWASyn_tiTrqSwaRtTime=0.2/1 -> Switch52/3
  Data Type Conversion52/1 -> Switch52/1, Switch52/2
  Data Type Conversion53/1 -> Switch53/2, Switch53/1
  LL_LKASWASyn_TrqSwaRateDiff=-0.2/1 -> Switch53/3
  Switch53/1 -> Bus Creator3/6  "LL_LKASWASyn_TrqSwaRateDiff"
  LL_LKAExPrcs_tiExitTime3=4/1 -> Switch54/3
  Data Type Conversion54/1 -> Switch54/1, Switch54/2
  Switch54/1 -> Bus Creator4/2  "LL_LKAExPrcs_tiExitTime2"
  Switch55/1 -> Bus Creator4/1  "LL_LKAExPrcs_tiExitTime1"
  Data Type Conversion55/1 -> Switch55/2, Switch55/1
  LL_LKAExPrcs_tiExitTime3=8/1 -> Switch55/3
  Switch9/1 -> Bus Creator2/12  "LL_LFClb_TFC_DiffCtlBalance"
  LL_LFClb_TFC_DiffCtlBalance=1.2/1 -> Switch9/3
  Data Type Conversion9/1 -> Switch9/1, Switch9/2
  [CLB_LKASWASyn_T2] -> Data Type Conversion24/1
  Switch16/1 -> Bus Creator3/10  "LL_LKASWASyn_T2"
  LL_LKASWASyn_T2=4/1 -> Switch16/3
  Data Type Conversion24/1 -> Switch16/1, Switch16/2
  Data Type Conversion20/1 -> Switch14/2, Switch14/1
  LL_LKASWASyn_M2=0.3/1 -> Switch14/3
  Switch14/1 -> Bus Creator3/9  "LL_LKASWASyn_M2"
  [CLB_LKASWASyn_M2] -> Data Type Conversion20/1
  [CLB_LKASWASyn_M1] -> Data Type Conversion19/1
  Switch13/1 -> Bus Creator3/8  "LL_LKASWASyn_M1"
  LL_LKASWASyn_M1=0.8/1 -> Switch13/3
  Data Type Conversion19/1 -> Switch13/1, Switch13/2
  Data Type Conversion12/1 -> Switch11/2, Switch11/1
  LL_LKASWASyn_M0=0.4/1 -> Switch11/3
  Switch11/1 -> Bus Creator3/7  "LL_LKASWASyn_M0"
  [CLB_LKASWASyn_M0] -> Data Type Conversion12/1
  Data Type Conversion25/1 -> Switch18/2, Switch18/1
  LL_LKASWASyn_M3K=0.2/1 -> Switch18/3
  Switch18/1 -> Bus Creator3/11  "LL_LKASWASyn_M3K"
  [CLB_LKASWASyn_M3K] -> Data Type Conversion25/1

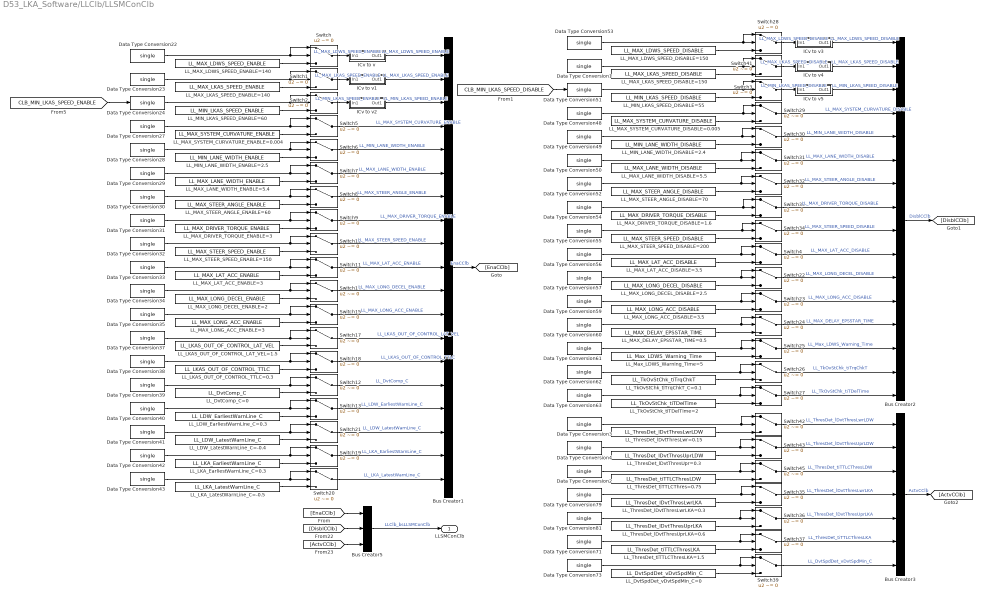
== system D53_LKA_Software/LLClb/LLSMConClb ==
  Bus Creator1 : BusCreator  Inputs=19
  Bus Creator2 : BusCreator  Inputs=16
  Bus Creator3 : BusCreator  Inputs=7
  Bus Creator5 : BusCreator  Inputs=3
  Data Type Conversion{1..4,22..24,27..35,37..43,48..57,59..63,71,73,79,81} (42 alike) : DataTypeConversion  OutDataTypeStr=single
  ICv to v : Subsystem
  ICv to v1 : Subsystem
  ICv to v2 : Subsystem
  ICv to v3 : Subsystem
  ICv to v4 : Subsystem
  ICv to v5 : Subsystem
  LL_DvtComp_C=0 : Constant  Value=LL_DvtComp_C  OutDataTypeStr=single
  LL_DvtSpdDet_vDvtSpdMin_C=0 : Constant  Value=LL_DvtSpdDet_vDvtSpdMin_C  OutDataTypeStr=single
  LL_LDW_EarliestWarnLine_C=0.3 : Constant  Value=LL_LDW_EarliestWarnLine_C  OutDataTypeStr=single
  LL_LDW_LatestWarnLine_C=-0.4 : Constant  Value=LL_LDW_LatestWarnLine_C  OutDataTypeStr=single
  LL_LKAS_OUT_OF_CONTROL_LAT_VEL=1.5 : Constant  Value=LL_LKAS_OUT_OF_CONTROL_LAT_VEL  OutDataTypeStr=single
  LL_LKAS_OUT_OF_CONTROL_TTLC=0.3 : Constant  Value=LL_LKAS_OUT_OF_CONTROL_TTLC  OutDataTypeStr=single
  LL_LKA_EarliestWarnLine_C=0.3 : Constant  Value=LL_LKA_EarliestWarnLine_C  OutDataTypeStr=single
  LL_LKA_LatestWarnLine_C=-0.5 : Constant  Value=LL_LKA_LatestWarnLine_C  OutDataTypeStr=single
  LL_MAX_DELAY_EPSSTAR_TIME=0.5 : Constant  Value=LL_MAX_DELAY_EPSSTAR_TIME  OutDataTypeStr=single
  LL_MAX_DRIVER_TORQUE_DISABLE=1.6 : Constant  Value=LL_MAX_DRIVER_TORQUE_DISABLE  OutDataTypeStr=single
  LL_MAX_DRIVER_TORQUE_ENABLE=3 : Constant  Value=LL_MAX_DRIVER_TORQUE_ENABLE  OutDataTypeStr=single
  LL_MAX_LANE_WIDTH_DISABLE=5.5 : Constant  Value=LL_MAX_LANE_WIDTH_DISABLE  OutDataTypeStr=single
  LL_MAX_LANE_WIDTH_ENABLE=5.4 : Constant  Value=LL_MAX_LANE_WIDTH_ENABLE  OutDataTypeStr=single
  LL_MAX_LAT_ACC_DISABLE=3.5 : Constant  Value=LL_MAX_LAT_ACC_DISABLE  OutDataTypeStr=single
  LL_MAX_LAT_ACC_ENABLE=3 : Constant  Value=LL_MAX_LAT_ACC_ENABLE  OutDataTypeStr=single
  LL_MAX_LDWS_SPEED_DISABLE=150 : Constant  Value=LL_MAX_LDWS_SPEED_DISABLE  OutDataTypeStr=single
  LL_MAX_LDWS_SPEED_ENABLE=140 : Constant  Value=LL_MAX_LDWS_SPEED_ENABLE  OutDataTypeStr=single
  LL_MAX_LKAS_SPEED_DISABLE=150 : Constant  Value=LL_MAX_LKAS_SPEED_DISABLE  OutDataTypeStr=single
  LL_MAX_LKAS_SPEED_ENABLE=140 : Constant  Value=LL_MAX_LKAS_SPEED_ENABLE  OutDataTypeStr=single
  LL_MAX_LONG_ACC_DISABLE=3.5 : Constant  Value=LL_MAX_LONG_ACC_DISABLE  OutDataTypeStr=single
  LL_MAX_LONG_ACC_ENABLE=3 : Constant  Value=LL_MAX_LONG_ACC_ENABLE  OutDataTypeStr=single
  LL_MAX_LONG_DECEL_DISABLE=2.5 : Constant  Value=LL_MAX_LONG_DECEL_DISABLE  OutDataTypeStr=single
  LL_MAX_LONG_DECEL_ENABLE=2 : Constant  Value=LL_MAX_LONG_DECEL_ENABLE  OutDataTypeStr=single
  LL_MAX_STEER_ANGLE_DISABLE=70 : Constant  Value=LL_MAX_STEER_ANGLE_DISABLE  OutDataTypeStr=single
  LL_MAX_STEER_ANGLE_ENABLE=60 : Constant  Value=LL_MAX_STEER_ANGLE_ENABLE  OutDataTypeStr=single
  LL_MAX_STEER_SPEED_DISABLE=200 : Constant  Value=LL_MAX_STEER_SPEED_DISABLE  OutDataTypeStr=single
  LL_MAX_STEER_SPEED_ENABLE=150 : Constant  Value=LL_MAX_STEER_SPEED_ENABLE  OutDataTypeStr=single
  LL_MAX_SYSTEM_CURVATURE_DISABLE=0.005 : Constant  Value=LL_MAX_SYSTEM_CURVATURE_DISABLE  OutDataTypeStr=single
  LL_MAX_SYSTEM_CURVATURE_ENABLE=0.004 : Constant  Value=LL_MAX_SYSTEM_CURVATURE_ENABLE  OutDataTypeStr=single
  LL_MIN_LANE_WIDTH_DISABLE=2.4 : Constant  Value=LL_MIN_LANE_WIDTH_DISABLE  OutDataTypeStr=single
  LL_MIN_LANE_WIDTH_ENABLE=2.5 : Constant  Value=LL_MIN_LANE_WIDTH_ENABLE  OutDataTypeStr=single
  LL_MIN_LKAS_SPEED_DISABLE=55 : Constant  Value=LL_MIN_LKAS_SPEED_DISABLE  OutDataTypeStr=single
  LL_MIN_LKAS_SPEED_ENABLE=60 : Constant  Value=LL_MIN_LKAS_SPEED_ENABLE  OutDataTypeStr=single
  LL_Max_LDWS_Warning_Time=5 : Constant  Value=LL_Max_LDWS_Warning_Time  OutDataTypeStr=single
  LL_ThresDet_lDvtThresLwr=0.15 : Constant  Value=LL_ThresDet_lDvtThresLwrLDW  OutDataTypeStr=single
  LL_ThresDet_lDvtThresLwrLKA=0.3 : Constant  Value=LL_ThresDet_lDvtThresLwrLKA  OutDataTypeStr=single
  LL_ThresDet_lDvtThresUpr=0.3 : Constant  Value=LL_ThresDet_lDvtThresUprLDW  OutDataTypeStr=single
  LL_ThresDet_lDvtThresUprLKA=0.6 : Constant  Value=LL_ThresDet_lDvtThresUprLKA  OutDataTypeStr=single
  LL_ThresDet_tiTTLCThres=0.75 : Constant  Value=LL_ThresDet_tiTTLCThresLDW  OutDataTypeStr=single
  LL_ThresDet_tiTTLCThresLKA=1.5 : Constant  Value=LL_ThresDet_tiTTLCThresLKA  OutDataTypeStr=single
  LL_TkOvStChk_tiTDelTime=2 : Constant  Value=LL_TkOvStChk_tiTDelTime  OutDataTypeStr=single
  LL_TkOvStChk_tiTrqChkT_C=0.1 : Constant  Value=LL_TkOvStChk_tiTrqChkT  OutDataTypeStr=single
  Switch{,1..15,17..37,39,41..43,45} (42 alike) : Switch  Criteria=u2 ~= 0  OutDataTypeStr=single
  LLSMConClb : Outport
  wires:
  Data Type Conversion39/1 -> Switch12/2, Switch12/1
  Switch10/1 -> Bus Creator1/9  "LL_MAX_STEER_SPEED_ENABLE"
  LL_MAX_LANE_WIDTH_ENABLE=5.4/1 -> Switch7/3
  Data Type Conversion42/1 -> Switch19/2, Switch19/1
  ICv to v2/1(Out1) -> Bus Creator1/3  "LL_MIN_LKAS_SPEED_ENABLE"
  LL_LKA_LatestWarnLine_C=-0.5/1 -> Switch20/3
  Data Type Conversion40/1 -> Switch13/2, Switch13/1
  LL_MAX_STEER_ANGLE_ENABLE=60/1 -> Switch8/3
  Data Type Conversion38/1 -> Switch18/2, Switch18/1
  Data Type Conversion43/1 -> Switch20/2, Switch20/1
  LL_MIN_LANE_WIDTH_ENABLE=2.5/1 -> Switch6/3
  Switch6/1 -> Bus Creator1/5  "LL_MIN_LANE_WIDTH_ENABLE"
  Switch17/1 -> Bus Creator1/13  "LL_LKAS_OUT_OF_CONTROL_LAT_VEL"
  LL_MAX_LONG_DECEL_ENABLE=2/1 -> Switch14/3
  Data Type Conversion30/1 -> Switch8/2, Switch8/1
  Data Type Conversion27/1 -> Switch5/2, Switch5/1
  Data Type Conversion31/1 -> Switch9/2, Switch9/1
  Data Type Conversion28/1 -> Switch6/2, Switch6/1
  LL_LKAS_OUT_OF_CONTROL_LAT_VEL=1.5/1 -> Switch17/3
  Data Type Conversion23/1 -> Switch1/2, Switch1/1
  LL_MIN_LKAS_SPEED_ENABLE=60/1 -> Switch2/3
  Data Type Conversion22/1 -> Switch/2, Switch/1
  Data Type Conversion24/1 -> Switch2/2, Switch2/1
  LL_MAX_LAT_ACC_ENABLE=3/1 -> Switch11/3
  LL_MAX_LDWS_SPEED_ENABLE=140/1 -> Switch/3
  Switch12/1 -> Bus Creator1/15  "LL_DvtComp_C"
  LL_LDW_LatestWarnLine_C=-0.4/1 -> Switch21/3
  Data Type Conversion29/1 -> Switch7/2, Switch7/1
  LL_MAX_LONG_ACC_ENABLE=3/1 -> Switch15/3
  LL_MAX_DRIVER_TORQUE_ENABLE=3/1 -> Switch9/3
  Data Type Conversion35/1 -> Switch15/2, Switch15/1
  LL_DvtComp_C=0/1 -> Switch12/3
  Switch19/1 -> Bus Creator1/18  "LL_LKA_EarliestWarnLine_C"
  LL_LKAS_OUT_OF_CONTROL_TTLC=0.3/1 -> Switch18/3
  Data Type Conversion32/1 -> Switch10/2, Switch10/1
  Data Type Conversion37/1 -> Switch17/2, Switch17/1
  Data Type Conversion33/1 -> Switch11/2, Switch11/1
  Switch7/1 -> Bus Creator1/6  "LL_MAX_LANE_WIDTH_ENABLE"
  Data Type Conversion34/1 -> Switch14/2, Switch14/1
  LL_LKA_EarliestWarnLine_C=0.3/1 -> Switch19/3
  Switch15/1 -> Bus Creator1/12  "LL_MAX_LONG_ACC_ENABLE"
  Switch18/1 -> Bus Creator1/14  "LL_LKAS_OUT_OF_CONTROL_TTLC"
  Switch21/1 -> Bus Creator1/17  "LL_LDW_LatestWarnLine_C"
  ICv to v/1(Out1) -> Bus Creator1/1  "LL_MAX_LDWS_SPEED_ENABLE"
  Switch20/1 -> Bus Creator1/19  "LL_LKA_LatestWarnLine_C"
  Switch14/1 -> Bus Creator1/11  "LL_MAX_LONG_DECEL_ENABLE"
  Switch13/1 -> Bus Creator1/16  "LL_LDW_EarliestWarnLine_C"
  Switch9/1 -> Bus Creator1/8  "LL_MAX_DRIVER_TORQUE_ENABLE"
  LL_MAX_STEER_SPEED_ENABLE=150/1 -> Switch10/3
  LL_MAX_SYSTEM_CURVATURE_ENABLE=0.004/1 -> Switch5/3
  Switch5/1 -> Bus Creator1/4  "LL_MAX_SYSTEM_CURVATURE_ENABLE"
  Switch8/1 -> Bus Creator1/7  "LL_MAX_STEER_ANGLE_ENABLE"
  Data Type Conversion41/1 -> Switch21/2, Switch21/1
  LL_LDW_EarliestWarnLine_C=0.3/1 -> Switch13/3
  ICv to v1/1(Out1) -> Bus Creator1/2  "LL_MAX_LKAS_SPEED_ENABLE"
  LL_MAX_LKAS_SPEED_ENABLE=140/1 -> Switch1/3
  Switch11/1 -> Bus Creator1/10  "LL_MAX_LAT_ACC_ENABLE"
  Data Type Conversion54/1 -> Switch33/2, Switch33/1
  Data Type Conversion63/1 -> Switch27/2, Switch27/1
  Data Type Conversion52/1 -> Switch32/2, Switch32/1
  Data Type Conversion61/1 -> Switch25/2, Switch25/1
  Switch26/1 -> Bus Creator2/15  "LL_TkOvStChk_tiTrqChkT"
  LL_MIN_LKAS_SPEED_DISABLE=55/1 -> Switch3/3
  Data Type Conversion60/1 -> Switch24/2, Switch24/1
  Data Type Conversion59/1 -> Switch23/2, Switch23/1
  Data Type Conversion49/1 -> Switch30/2, Switch30/1
  Switch30/1 -> Bus Creator2/5  "LL_MIN_LANE_WIDTH_DISABLE"
  Data Type Conversion62/1 -> Switch26/2, Switch26/1
  LL_MAX_LONG_DECEL_DISABLE=2.5/1 -> Switch22/3
  Switch25/1 -> Bus Creator2/14  "LL_Max_LDWS_Warning_Time"
  Data Type Conversion57/1 -> Switch22/1, Switch22/2
  Switch29/1 -> Bus Creator2/4  "LL_MAX_SYSTEM_CURVATURE_DISABLE"
  Data Type Conversion48/1 -> Switch29/2, Switch29/1
  LL_MAX_SYSTEM_CURVATURE_DISABLE=0.005/1 -> Switch29/3
  Switch23/1 -> Bus Creator2/12  "LL_MAX_LONG_ACC_DISABLE"
  LL_MAX_DELAY_EPSSTAR_TIME=0.5/1 -> Switch24/3
  Data Type Conversion53/1 -> Switch28/2, Switch28/1
  LL_MAX_DRIVER_TORQUE_DISABLE=1.6/1 -> Switch33/3
  LL_MAX_LANE_WIDTH_DISABLE=5.5/1 -> Switch31/3
  LL_TkOvStChk_tiTrqChkT_C=0.1/1 -> Switch26/3
  LL_MAX_LDWS_SPEED_DISABLE=150/1 -> Switch28/3
  Switch4/1 -> Bus Creator2/10  "LL_MAX_LAT_ACC_DISABLE"
  Data Type Conversion50/1 -> Switch31/2, Switch31/1
  Data Type Conversion51/1 -> Switch3/1, Switch3/2
  LL_MAX_LAT_ACC_DISABLE=3.5/1 -> Switch4/3
  Data Type Conversion55/1 -> Switch34/2, Switch34/1
  Switch33/1 -> Bus Creator2/8  "LL_MAX_DRIVER_TORQUE_DISABLE"
  LL_MIN_LANE_WIDTH_DISABLE=2.4/1 -> Switch30/3
  LL_Max_LDWS_Warning_Time=5/1 -> Switch25/3
  LL_MAX_STEER_SPEED_DISABLE=200/1 -> Switch34/3
  LL_MAX_LONG_ACC_DISABLE=3.5/1 -> Switch23/3
  Switch22/1 -> Bus Creator2/11  "LL_MAX_LONG_DECEL_DISABLE"
  Switch24/1 -> Bus Creator2/13  "LL_MAX_DELAY_EPSSTAR_TIME"
  Switch32/1 -> Bus Creator2/7  "LL_MAX_STEER_ANGLE_DISABLE"
  Switch34/1 -> Bus Creator2/9  "LL_MAX_STEER_SPEED_DISABLE"
  Switch31/1 -> Bus Creator2/6  "LL_MAX_LANE_WIDTH_DISABLE"
  Data Type Conversion56/1 -> Switch4/1, Switch4/2
  LL_MAX_STEER_ANGLE_DISABLE=70/1 -> Switch32/3
  ICv to v5/1(Out1) -> Bus Creator2/3  "LL_MIN_LKAS_SPEED_DISABLE"
  LL_TkOvStChk_tiTDelTime=2/1 -> Switch27/3
  Switch27/1 -> Bus Creator2/16  "LL_TkOvStChk_tiTDelTime"
  Bus Creator2/1 -> [DisblCClb]  "DisblCClb"
  Data Type Conversion81/1 -> Switch36/2, Switch36/1
  LL_ThresDet_tiTTLCThresLKA=1.5/1 -> Switch37/3
  LL_DvtSpdDet_vDvtSpdMin_C=0/1 -> Switch39/3
  Data Type Conversion71/1 -> Switch37/2, Switch37/1
  LL_ThresDet_lDvtThresLwrLKA=0.3/1 -> Switch35/3
  Data Type Conversion79/1 -> Switch35/1, Switch35/2
  LL_ThresDet_lDvtThresUprLKA=0.6/1 -> Switch36/3
  Switch39/1 -> Bus Creator3/7  "LL_DvtSpdDet_vDvtSpdMin_C"
  Switch37/1 -> Bus Creator3/6  "LL_ThresDet_tiTTLCThresLKA"
  Switch35/1 -> Bus Creator3/4  "LL_ThresDet_lDvtThresLwrLKA"
  Switch36/1 -> Bus Creator3/5  "LL_ThresDet_lDvtThresUprLKA"
  Data Type Conversion73/1 -> Switch39/1, Switch39/2
  Bus Creator1/1 -> [EnaCClb]  "EnaCClb"
  Bus Creator3/1 -> [ActvCClb]  "ActvCClb"
  [EnaCClb] -> Bus Creator5/1
  [DisblCClb] -> Bus Creator5/2
  [ActvCClb] -> Bus Creator5/3
  Bus Creator5/1 -> LLSMConClb/1  "LLClb_bsLLSMConClb"
  ICv to v4/1(Out1) -> Bus Creator2/2  "LL_MAX_LKAS_SPEED_DISABLE"
  Data Type Conversion1/1 -> Switch41/2, Switch41/1
  LL_MAX_LKAS_SPEED_DISABLE=150/1 -> Switch41/3
  Switch43/1 -> Bus Creator3/2  "LL_ThresDet_lDvtThresUprLDW"
  Switch42/1 -> Bus Creator3/1  "LL_ThresDet_lDvtThresLwrLDW"
  Switch45/1 -> Bus Creator3/3  "LL_ThresDet_tiTTLCThresLDW"
  LL_ThresDet_lDvtThresUpr=0.3/1 -> Switch43/3
  Data Type Conversion3/1 -> Switch42/2, Switch42/1
  LL_ThresDet_lDvtThresLwr=0.15/1 -> Switch42/3
  Data Type Conversion2/1 -> Switch45/1, Switch45/2
  LL_ThresDet_tiTTLCThres=0.75/1 -> Switch45/3
  Data Type Conversion4/1 -> Switch43/1, Switch43/2
  Switch/1 -> ICv to v/1(In1)  "LL_MAX_LDWS_SPEED_ENABLE"
  Switch1/1 -> ICv to v1/1(In1)  "LL_MAX_LKAS_SPEED_ENABLE"
  Switch2/1 -> ICv to v2/1(In1)  "LL_MIN_LKAS_SPEED_ENABLE"
  Switch28/1 -> ICv to v3/1(In1)  "LL_MAX_LDWS_SPEED_DISABLE"
  ICv to v3/1(Out1) -> Bus Creator2/1  "LL_MAX_LDWS_SPEED_DISABLE"
  Switch41/1 -> ICv to v4/1(In1)  "LL_MAX_LKAS_SPEED_DISABLE"
  Switch3/1 -> ICv to v5/1(In1)  "LL_MIN_LKAS_SPEED_DISABLE"
  [CLB_MIN_LKAS_SPEED_ENABLE] -> Data Type Conversion24/1
  [CLB_MIN_LKAS_SPEED_DISABLE] -> Data Type Conversion51/1

== system D53_LKA_Software/LLClb_bsLLClb_Read_Num=100/Subsystem1 ==
  CAN Unpack : canmsglib/CAN Unpack  MsgList=(none)  MsgName=CAN Msg  MsgIDType=Extended (29-bit identifier)  MsgIdentifier=120534787  MsgLength=8  SignalInfo=Serial number$0$8$1$2$1$0$1$0$-Inf$Inf$#index$8$8$1$2$1$0$1$-100$-Inf$Inf$#coefficient$16$32$1$2$1$0$0.000001$-10$-Inf$Inf$#  NSignals=3  IDPort=off  TimestampPort=off  ErrorPort=off  RemotePort=off  LengthPort=off  StatusPort=off  StartBits=str2num('[int32(0);int32(8);int32(16)]')  SignalSizes=str2num('[int32(8);int32(8);int32(32)]')  ByteOrders=str2num('[int32(1);int32(1);int32(1)]')  DataTypes=str2num('[int32(2);int32(2);int32(2)]')  MultiplexTypes=str2num('[int32(1);int32(1);int32(1)]')  MultiplexValues=str2num('[double(0);double(0);double(0)]')  Factors=str2num('[double(1);double(1);double(0.000001)]')  Offsets=str2num('[double(0);double(-100);double(-10)]')  Minimums=str2num('[double(-Inf);double(-Inf);double(-Inf)]')  Maximums=str2num('[double(Inf);double(Inf);double(Inf)]')  ApplyMinMax=off
      settings: SourceProductName=Simulink Real-Time  SourceProductBaseCode=XP
  S-Function2 : S-Function  FunctionName=CAN_Rec_P  Parameters=uint8(Module-1),uint32(ID),uint8(Frameformat-1),uint8(Newflag),uint8(FIFO),double(sampletime)  SFunctionDeploymentMode=off  EnableBusSupport=off  mask(CAN_receive){Module=CAN_0, ID=120534787, Frameformat=Extended (29-bit identifier), Newflag=on, FIFO=off, sampletime=0.01}
      mask prompts: Module "CAN Port:"; ID "CAN Frame ID:"; Frameformat "CAN Frame Format:"; FIFO "Overflow flag"
      mask init:
      | maskdisplay = canrecicon(Module,ID,Frameformat,Newflag,FIFO);
      | set_param(gcb, 'MaskDisplay', maskdisplay);
      mask TypeOptions Module: CAN_0 | CAN_1 | CAN_2 | CAN_3
      mask TypeOptions Frameformat: Standard (11-bit identifier) | Extended (29-bit identifier)
      mask Display: color('blue');text(0.98,0.9,'MPC5675K','horizontalAlignment','right');color('black');text(0.5,0.6,'FlexCAN_0 Receive','horizontalAlignment','center');text(0.5,0.35,'Extended ID:120534787','horizontalAlignment','center');port_label('output',1,'New_Flag');port_label('output',2,'CAN_Msg');
  Out1 : Outport
  Out2 : Outport  Port=2
  Out3 : Outport  Port=3
  wires:
  S-Function2/2 -> CAN Unpack/1
  CAN Unpack/1 -> Out1/1
  CAN Unpack/2 -> Out2/1
  CAN Unpack/3 -> Out3/1
